simulink model "LCK"  (R2018b)
settings: Solver=FixedStepDiscrete  StartTime=0.0  StopTime=inf  FixedStep=0.01  RelTol=1e-3
PostLoadFcn:
  | if any(exist('dsrtsu_mdlpostloadfcn', 'file') ~= 0), dsrtsu_mdlpostloadfcn('Execute', bdroot); end
values from neighbouring files (symbols this model uses):
  C_DEG2RAD = 0.0175    [LCK_Macro.sldd]
  C_KPH2MPS = 0.2778    [LCK_Macro.sldd]
  C_NEARZERO = 0.0001    [LCK_Macro.sldd]
  C_ONE = 1.0    [LCK_Macro.sldd]
  C_RAD2DEG = 57.2958    [LCK_Macro.sldd]
  C_ZERO = 0.0    [LCK_Macro.sldd]
  k_accel_pedal_pos_per_speed_x : value not decoded    [LCK_LogicPara.sldd]
  k_accel_pedal_pos_per_speed_z : value not decoded    [LCK_LogicPara.sldd]
  k_brake_suprress_hold = 1000.0    [LCK_LogicPara.sldd]
  k_driver_appl_torque_filt = 50.0    [LCK_LogicPara.sldd]
  k_driver_suppression_hold_time = 3000.0    [LCK_LogicPara.sldd]
  k_hands_on_wheel_hold_msec = 500.0    [LCK_LogicPara.sldd]
  k_hands_on_wheel_torque_hi = 0.2    [LCK_LogicPara.sldd]
  k_hands_on_wheel_torque_lo = 0.15    [LCK_LogicPara.sldd]
  k_handsoff_delay_cycles = 50.0    [LCK_LogicPara.sldd]
  k_handsoff_torq_Lo_CR = 0.3    [LCK_LogicPara.sldd]
  k_handson_delay_cycles = 5.0    [LCK_LogicPara.sldd]
  k_HighAccel_suppress_hold = 3000.0    [LCK_LogicPara.sldd]
  k_HLR_suprress_hold = 3000.0    [LCK_LogicPara.sldd]
  k_hs_StrAng_CR_threshold_z : value not decoded    [LCK_LogicPara.sldd]
  k_LC_Exit_Switch = 0.0    [LCK_LogicPara.sldd]
  k_LCG_Configured = 1.0    [LCK_LogicPara.sldd]
  k_LCK_A0_Rdy2Act_UseConst = 0.0    [LCK_LogicPara.sldd]
  k_LCK_A0Fac_ActSta : value not decoded    [LCK_CtrlPara.sldd]
  k_LCK_A0Fac_DrvStm : value not decoded    [LCK_CtrlPara.sldd]
  k_LCK_A0Shift_LftCurv : value not decoded    [LCK_CtrlPara.sldd]
  k_LCK_A0Shift_RgtCurv : value not decoded    [LCK_CtrlPara.sldd]
  k_LCK_A0Shift_StraLan = 0.0    [LCK_CtrlPara.sldd]
  k_LCK_A0ShiftFac_Dy_LftCurv : value not decoded    [LCK_CtrlPara.sldd]
  k_LCK_A0ShiftFac_Dy_RgtCurv : value not decoded    [LCK_CtrlPara.sldd]
  k_LCK_A0ShiftFac_Vspd : value not decoded    [LCK_CtrlPara.sldd]
  k_LCK_accel_inhibit_thold = 35.0    [LCK_LogicPara.sldd]
  k_LCK_Active2Ready_Mask = 255.0    [LCK_LogicPara.sldd]
  k_LCK_CvatRateBks : value not decoded    [LCK_CtrlPara.sldd]
  k_LCK_CvatrBks : value not decoded    [LCK_CtrlPara.sldd]
  k_LCK_DFac_Dy : value not decoded    [LCK_CtrlPara.sldd]
  k_LCK_DFac_Dy_Curv : value not decoded    [LCK_CtrlPara.sldd]
  k_LCK_DFac_HaCurCen : value not decoded    [LCK_CtrlPara.sldd]
  k_LCK_DFac_HaCurSid : value not decoded    [LCK_CtrlPara.sldd]
  k_LCK_DFac_HadCurCen : value not decoded    [LCK_CtrlPara.sldd]
  k_LCK_DFac_HadCurSid : value not decoded    [LCK_CtrlPara.sldd]
  k_LCK_DFac_HadStrCen : value not decoded    [LCK_CtrlPara.sldd]
  k_LCK_DFac_HadStrSid : value not decoded    [LCK_CtrlPara.sldd]
  k_LCK_DFac_HaStrCen : value not decoded    [LCK_CtrlPara.sldd]
  k_LCK_DFac_HaStrSid : value not decoded    [LCK_CtrlPara.sldd]
  k_LCK_DFac_Rad : value not decoded    [LCK_CtrlPara.sldd]
  k_LCK_DFac_SA_CurCen : value not decoded    [LCK_CtrlPara.sldd]
  k_LCK_DFac_SA_CurSid : value not decoded    [LCK_CtrlPara.sldd]
  k_LCK_DFac_SA_StrCen : value not decoded    [LCK_CtrlPara.sldd]
  k_LCK_DFac_SA_StrSid : value not decoded    [LCK_CtrlPara.sldd]
  k_LCK_DFac_SS_CurCen : value not decoded    [LCK_CtrlPara.sldd]
  k_LCK_DFac_SS_CurSid : value not decoded    [LCK_CtrlPara.sldd]
  k_LCK_DFac_SS_StrCen : value not decoded    [LCK_CtrlPara.sldd]
  k_LCK_DFac_SS_StrSid : value not decoded    [LCK_CtrlPara.sldd]
  k_LCK_DFac_Vspd : value not decoded    [LCK_CtrlPara.sldd]
  k_LCK_DlyTm_DrvStim = 0.2    [LCK_CtrlPara.sldd]
  k_LCK_DTermMax = 2.0    [LCK_CtrlPara.sldd]
  k_LCK_DyBks_Curv : value not decoded    [LCK_CtrlPara.sldd]
  k_LCK_Enable_POOnly = 1.0    [LCK_LogicPara.sldd]
  k_LCK_Entry_DistBuffer = 0.1    [LCK_LogicPara.sldd]
  k_LCK_Fac_Vspd2RngThr_FalRec = 0.23    [LCK_CtrlPara.sldd]
  k_LCK_Ffw_CvatSwh = 0.0    [LCK_CtrlPara.sldd]
  k_LCK_Ffw_DyBks : value not decoded    [LCK_CtrlPara.sldd]
  k_LCK_Ffw_TimCon_CmdFlt = 0.0    [LCK_CtrlPara.sldd]
  k_LCK_FfwDeltaFac_Rad_Lft : value not decoded    [LCK_CtrlPara.sldd]
  k_LCK_FfwDeltaFac_Rad_Rgt : value not decoded    [LCK_CtrlPara.sldd]
  k_LCK_FfwDeltaFac_Vspd : value not decoded    [LCK_CtrlPara.sldd]
  k_LCK_FfwFac_CvatRate_Lft : value not decoded    [LCK_CtrlPara.sldd]
  k_LCK_FfwFac_CvatRate_Rgt : value not decoded    [LCK_CtrlPara.sldd]
  k_LCK_FfwFac_Dy : value not decoded    [LCK_CtrlPara.sldd]
  k_LCK_FfwFac_Rad_Lft : value not decoded    [LCK_CtrlPara.sldd]
  k_LCK_FfwFac_Rad_Rgt : value not decoded    [LCK_CtrlPara.sldd]
  k_LCK_FfwFac_Vspd : value not decoded    [LCK_CtrlPara.sldd]
  k_LCK_FfwTorq_Cvat : value not decoded    [LCK_CtrlPara.sldd]
  k_LCK_HAFac_ActSta : value not decoded    [LCK_CtrlPara.sldd]
  k_LCK_HAFac_DrvStm : value not decoded    [LCK_CtrlPara.sldd]
  k_LCK_HaloTime = 2000.0    [LCK_LogicPara.sldd]
  k_LCK_HaloTime_Switch = 0.0    [LCK_LogicPara.sldd]
  k_LCK_HARFac_ActSta : value not decoded    [LCK_CtrlPara.sldd]
  k_LCK_HARFac_DrvStm : value not decoded    [LCK_CtrlPara.sldd]
  k_LCK_Hed_DyBks : value not decoded    [LCK_CtrlPara.sldd]
  k_LCK_HedAngDiffX : value not decoded    [LCK_CtrlPara.sldd]
  k_LCK_HedAngRateDiffX : value not decoded    [LCK_CtrlPara.sldd]
  k_LCK_HndsOnWhel_DlyTm_Idl2Rdy = 0.0    [LCK_LogicPara.sldd]
  k_LCK_host_veh_width = 1.86    [LCK_LogicPara.sldd]
  k_LCK_Idle2Ready_Mask = 239.0    [LCK_LogicPara.sldd]
  k_LCK_Junc_SusTime = 1.0    [LCK_LogicPara.sldd]
  k_LCK_KpKdDecSlopeLmt = 10.0    [LCK_CtrlPara.sldd]
  k_LCK_KpKdIncSlopeLmt = 5.0    [LCK_CtrlPara.sldd]
  k_LCK_Lat_Ctrl_DFac_Lft = 1.0    [LCK_CtrlPara.sldd]
  k_LCK_Lat_Ctrl_DFac_Rgt = 1.05    [LCK_CtrlPara.sldd]
  k_LCK_Lat_Ctrl_Kd = 0.8    [LCK_CtrlPara.sldd]
  k_LCK_Lat_Ctrl_Ki = 0.5    [LCK_CtrlPara.sldd]
  k_LCK_Lat_Ctrl_Kp = 0.7    [LCK_CtrlPara.sldd]
  k_LCK_Lat_Ctrl_Kp_NearGain = 0.7    [LCK_CtrlPara.sldd]
  k_LCK_Lat_Ctrl_PFac_Lft = 1.0    [LCK_CtrlPara.sldd]
  k_LCK_Lat_Ctrl_PFac_Rgt = 1.05    [LCK_CtrlPara.sldd]
  k_LCK_Lat_Ctrl_TimCon_CmdFlt = 5.0    [LCK_CtrlPara.sldd]
  k_LCK_Lat_DFac_Rad : value not decoded    [LCK_CtrlPara.sldd]
  k_LCK_Lat_DFac_SS_Cur : value not decoded    [LCK_CtrlPara.sldd]
  k_LCK_Lat_DFac_SS_Str : value not decoded    [LCK_CtrlPara.sldd]
  k_LCK_Lat_DFac_Vspd : value not decoded    [LCK_CtrlPara.sldd]
  k_LCK_Lat_DyBks : value not decoded    [LCK_CtrlPara.sldd]
  k_LCK_Lat_IFac_Rad : value not decoded    [LCK_CtrlPara.sldd]
  k_LCK_Lat_IFac_Vspd : value not decoded    [LCK_CtrlPara.sldd]
  k_LCK_Lat_ILmtFac_Dy_CurvLan : value not decoded    [LCK_CtrlPara.sldd]
  k_LCK_Lat_ILmtFac_Dy_StraLan : value not decoded    [LCK_CtrlPara.sldd]
  k_LCK_Lat_ILmtFac_Rad : value not decoded    [LCK_CtrlPara.sldd]
  k_LCK_Lat_ILmtFac_Rad_NearGain = 1.0    [LCK_CtrlPara.sldd]
  k_LCK_Lat_ILmtFac_Vspd_CurvLan : value not decoded    [LCK_CtrlPara.sldd]
  k_LCK_Lat_ILmtFac_Vspd_StraLan : value not decoded    [LCK_CtrlPara.sldd]
  k_LCK_Lat_ITermLmt_Dy = 1.0    [LCK_CtrlPara.sldd]
  k_LCK_Lat_KpKdDecSlopeLmt = 10.0    [LCK_CtrlPara.sldd]
  k_LCK_Lat_KpKdIncSlopeLmt = 10.0    [LCK_CtrlPara.sldd]
  k_LCK_Lat_PFac_Dy_InnLftCur : value not decoded    [LCK_CtrlPara.sldd]
  k_LCK_Lat_PFac_Dy_InnRgtCur : value not decoded    [LCK_CtrlPara.sldd]
  k_LCK_Lat_PFac_Dy_OutLftCur : value not decoded    [LCK_CtrlPara.sldd]
  k_LCK_Lat_PFac_Dy_OutRgtCur : value not decoded    [LCK_CtrlPara.sldd]
  k_LCK_Lat_PFac_Dy_Str : value not decoded    [LCK_CtrlPara.sldd]
  k_LCK_Lat_PFac_Rad : value not decoded    [LCK_CtrlPara.sldd]
  ... (+153 more)
undefined symbols (not defined in the file or in its folder): k_LCK_CurvBks, K_LCK_SPA0A1A2_LMRngCmp_y
libraries: LateralControl_fcns_lib x59, simulink x24
(part 38 of 47)

== system LCK/Lateral_Control_Module/Adas_Lateral_Control_LCK_Core/Module 8/Module 0/Definition  Limit ==
  Road_Radius : Inport
  Vspd : Inport  Port=2
  Dy_1 : Inport  Port=3
  Str_Flag : Inport  Port=4
  Abs : Abs
  Add : Sum
  Constant : Constant  OutDataTypeStr=single
  Divide : Product  Inputs=*/
  Product1 : Product  Inputs=4
  Product2 : Product  Inputs=4
  Product7 : Product
  Switch4 : Switch  Criteria=u2 > Threshold
  Switch5 : Switch  Criteria=u2 > Threshold
  k_LCK_Lat_ILmtFac_Dy_CurvLan : Lookup_n-D  NumberOfTableDimensions=1  BreakpointsForDimension1=k_LCK_Lat_DyBks  IndexSearchMethod=Linear search  Table=k_LCK_Lat_ILmtFac_Dy_CurvLan  ExtrapMethod=Clip  InternalRulePriority=Speed  RndMeth=Simplest  InputSameDT=on
  k_LCK_Lat_ILmtFac_Dy_StraLan : Lookup_n-D  NumberOfTableDimensions=1  BreakpointsForDimension1=k_LCK_Lat_DyBks  IndexSearchMethod=Linear search  Table=k_LCK_Lat_ILmtFac_Dy_StraLan  ExtrapMethod=Clip  InternalRulePriority=Speed  RndMeth=Simplest  InputSameDT=on
  k_LCK_Lat_ILmtFac_Rad : Lookup_n-D  NumberOfTableDimensions=1  BreakpointsForDimension1=k_LCK_RadBks  IndexSearchMethod=Linear search  Table=k_LCK_Lat_ILmtFac_Rad  ExtrapMethod=Clip  InternalRulePriority=Speed  RndMeth=Simplest  InputSameDT=on
  k_LCK_Lat_ILmtFac_Rad_NearGain : Constant  Value=k_LCK_Lat_ILmtFac_Rad_NearGain
  k_LCK_Lat_ILmtFac_Vspd_CurvLan : Lookup_n-D  NumberOfTableDimensions=1  BreakpointsForDimension1=k_LCK_VspdBks  IndexSearchMethod=Linear search  Table=k_LCK_Lat_ILmtFac_Vspd_CurvLan  ExtrapMethod=Clip  InternalRulePriority=Speed  RndMeth=Simplest  InputSameDT=on
  k_LCK_Lat_ILmtFac_Vspd_StraLan : Lookup_n-D  NumberOfTableDimensions=1  BreakpointsForDimension1=k_LCK_VspdBks  IndexSearchMethod=Linear search  Table=k_LCK_Lat_ILmtFac_Vspd_StraLan  ExtrapMethod=Clip  InternalRulePriority=Speed  RndMeth=Simplest  InputSameDT=on
  k_LCK_Lat_ITermLmt_Dy : Constant  Value=k_LCK_Lat_ITermLmt_Dy
  ITerm_Limit_1 : Outport
  ITerm_Limit_0 : Outport  Port=2
  wires:
  Vspd/1 -> k_LCK_Lat_ILmtFac_Vspd_CurvLan/1, k_LCK_Lat_ILmtFac_Vspd_StraLan/1
  k_LCK_Lat_ILmtFac_Vspd_CurvLan/1 -> Switch5/3
  Str_Flag/1 -> Switch5/2, Switch4/2
  k_LCK_Lat_ILmtFac_Vspd_StraLan/1 -> Switch5/1
  k_LCK_Lat_ILmtFac_Dy_CurvLan/1 -> Switch4/3
  k_LCK_Lat_ILmtFac_Dy_StraLan/1 -> Switch4/1
  Road_Radius/1 -> k_LCK_Lat_ILmtFac_Rad/1
  Dy_1/1 -> Abs/1
  Switch4/1 -> Product2/2, Product1/1
  Switch5/1 -> Product2/3, Product1/2
  k_LCK_Lat_ITermLmt_Dy/1 -> Product2/1, Product1/4
  Product2/1 -> ITerm_Limit_0/1
  Product1/1 -> ITerm_Limit_1/1
  Abs/1 -> k_LCK_Lat_ILmtFac_Dy_StraLan/1, k_LCK_Lat_ILmtFac_Dy_CurvLan/1
  k_LCK_Lat_ILmtFac_Rad_NearGain/1 -> Product7/2, Add/2
  Constant/1 -> Add/1
  k_LCK_Lat_ILmtFac_Rad/1 -> Divide/1
  Add/1 -> Divide/2
  Divide/1 -> Product1/3, Product7/1
  Product7/1 -> Product2/4

== system LCK/Lateral_Control_Module/Adas_Lateral_Control_LCK_Core/Module 8/Module 0/Definition Fac 2 ==
  Dy_0 : Inport
  Str_Flag : Inport  Port=2
  Inn_Cur_Flag_0 : Inport  Port=3
  Cur_Flag : Inport  Port=4
  Abs : Abs
  Switch{3,10,12..13} (4 alike) : Switch  Criteria=u2 > Threshold
  k_LCK_Lat_PFac_Dy_InnLftCur : Lookup_n-D  NumberOfTableDimensions=1  BreakpointsForDimension1=k_LCK_Lat_DyBks  IndexSearchMethod=Linear search  Table=k_LCK_Lat_PFac_Dy_InnLftCur  ExtrapMethod=Clip  InternalRulePriority=Speed  RndMeth=Simplest  InputSameDT=on
  k_LCK_Lat_PFac_Dy_InnRgtCur : Lookup_n-D  NumberOfTableDimensions=1  BreakpointsForDimension1=k_LCK_Lat_DyBks  IndexSearchMethod=Linear search  Table=k_LCK_Lat_PFac_Dy_InnRgtCur  ExtrapMethod=Clip  InternalRulePriority=Speed  RndMeth=Simplest  InputSameDT=on
  k_LCK_Lat_PFac_Dy_OutLftCur : Lookup_n-D  NumberOfTableDimensions=1  BreakpointsForDimension1=k_LCK_Lat_DyBks  IndexSearchMethod=Linear search  Table=k_LCK_Lat_PFac_Dy_OutLftCur  ExtrapMethod=Clip  InternalRulePriority=Speed  RndMeth=Simplest  InputSameDT=on
  k_LCK_Lat_PFac_Dy_OutRgtCur : Lookup_n-D  NumberOfTableDimensions=1  BreakpointsForDimension1=k_LCK_Lat_DyBks  IndexSearchMethod=Linear search  Table=k_LCK_Lat_PFac_Dy_OutRgtCur  ExtrapMethod=Clip  InternalRulePriority=Speed  RndMeth=Simplest  InputSameDT=on
  k_LCK_Lat_PFac_Dy_Str : Lookup_n-D  NumberOfTableDimensions=1  BreakpointsForDimension1=k_LCK_Lat_DyBks  IndexSearchMethod=Linear search  Table=k_LCK_Lat_PFac_Dy_Str  ExtrapMethod=Clip  InternalRulePriority=Speed  RndMeth=Simplest  InputSameDT=on
  LatCtrl_P0Fac_Dy : Outport
  wires:
  k_LCK_Lat_PFac_Dy_OutLftCur/1 -> Switch10/3
  Inn_Cur_Flag_0/1 -> Switch13/2, Switch10/2
  k_LCK_Lat_PFac_Dy_InnLftCur/1 -> Switch10/1
  Switch10/1 -> Switch12/1
  Switch13/1 -> Switch12/3
  Dy_0/1 -> Abs/1
  Switch12/1 -> Switch3/3
  Cur_Flag/1 -> Switch12/2
  k_LCK_Lat_PFac_Dy_OutRgtCur/1 -> Switch13/3
  k_LCK_Lat_PFac_Dy_InnRgtCur/1 -> Switch13/1
  k_LCK_Lat_PFac_Dy_Str/1 -> Switch3/1
  Str_Flag/1 -> Switch3/2
  Switch3/1 -> LatCtrl_P0Fac_Dy/1
  Abs/1 -> k_LCK_Lat_PFac_Dy_Str/1, k_LCK_Lat_PFac_Dy_OutRgtCur/1, k_LCK_Lat_PFac_Dy_InnRgtCur/1, k_LCK_Lat_PFac_Dy_OutLftCur/1, k_LCK_Lat_PFac_Dy_InnLftCur/1

== system LCK/Lateral_Control_Module/Adas_Lateral_Control_LCK_Core/Module 8/Module 0/Definition Fac 3 ==
  Cur_Flag : Inport
  Inn_Cur_Flag_1 : Inport  Port=2
  Dy_1 : Inport  Port=3
  Str_Flag : Inport  Port=4
  Abs : Abs
  Switch{3,10,12..13} (4 alike) : Switch  Criteria=u2 > Threshold
  k_LCK_Lat_PFac_Dy_InnLftCur : Lookup_n-D  NumberOfTableDimensions=1  BreakpointsForDimension1=k_LCK_Lat_DyBks  IndexSearchMethod=Linear search  Table=k_LCK_Lat_PFac_Dy_InnLftCur  ExtrapMethod=Clip  InternalRulePriority=Speed  RndMeth=Simplest  InputSameDT=on
  k_LCK_Lat_PFac_Dy_InnRgtCur : Lookup_n-D  NumberOfTableDimensions=1  BreakpointsForDimension1=k_LCK_Lat_DyBks  IndexSearchMethod=Linear search  Table=k_LCK_Lat_PFac_Dy_InnRgtCur  ExtrapMethod=Clip  InternalRulePriority=Speed  RndMeth=Simplest  InputSameDT=on
  k_LCK_Lat_PFac_Dy_OutLftCur : Lookup_n-D  NumberOfTableDimensions=1  BreakpointsForDimension1=k_LCK_Lat_DyBks  IndexSearchMethod=Linear search  Table=k_LCK_Lat_PFac_Dy_OutLftCur  ExtrapMethod=Clip  InternalRulePriority=Speed  RndMeth=Simplest  InputSameDT=on
  k_LCK_Lat_PFac_Dy_OutRgtCur : Lookup_n-D  NumberOfTableDimensions=1  BreakpointsForDimension1=k_LCK_Lat_DyBks  IndexSearchMethod=Linear search  Table=k_LCK_Lat_PFac_Dy_OutRgtCur  ExtrapMethod=Clip  InternalRulePriority=Speed  RndMeth=Simplest  InputSameDT=on
  k_LCK_Lat_PFac_Dy_Str : Lookup_n-D  NumberOfTableDimensions=1  BreakpointsForDimension1=k_LCK_Lat_DyBks  IndexSearchMethod=Linear search  Table=k_LCK_Lat_PFac_Dy_Str  ExtrapMethod=Clip  InternalRulePriority=Speed  RndMeth=Simplest  InputSameDT=on
  LatCtrl_P1Fac_Dy : Outport
  wires:
  Abs/1 -> k_LCK_Lat_PFac_Dy_InnLftCur/1, k_LCK_Lat_PFac_Dy_OutLftCur/1, k_LCK_Lat_PFac_Dy_InnRgtCur/1, k_LCK_Lat_PFac_Dy_OutRgtCur/1, k_LCK_Lat_PFac_Dy_Str/1
  Switch3/1 -> LatCtrl_P1Fac_Dy/1
  Str_Flag/1 -> Switch3/2
  k_LCK_Lat_PFac_Dy_Str/1 -> Switch3/1
  k_LCK_Lat_PFac_Dy_InnRgtCur/1 -> Switch13/1
  k_LCK_Lat_PFac_Dy_OutRgtCur/1 -> Switch13/3
  Cur_Flag/1 -> Switch12/2
  Switch12/1 -> Switch3/3
  Dy_1/1 -> Abs/1
  Switch13/1 -> Switch12/3
  Switch10/1 -> Switch12/1
  k_LCK_Lat_PFac_Dy_InnLftCur/1 -> Switch10/1
  Inn_Cur_Flag_1/1 -> Switch10/2, Switch13/2
  k_LCK_Lat_PFac_Dy_OutLftCur/1 -> Switch10/3

== system LCK/Lateral_Control_Module/Adas_Lateral_Control_LCK_Core/Module 8/Module 0/Definition Fac 4 ==
  Vspd : Inport
  k_LCK_Lat_DFac_Vspd : Lookup_n-D  NumberOfTableDimensions=1  BreakpointsForDimension1=k_LCK_VspdBks  IndexSearchMethod=Linear search  Table=k_LCK_Lat_DFac_Vspd  ExtrapMethod=Clip  InternalRulePriority=Speed  RndMeth=Simplest  InputSameDT=on
  k_LCK_Lat_IFac_Vspd : Lookup_n-D  NumberOfTableDimensions=1  BreakpointsForDimension1=k_LCK_VspdBks  IndexSearchMethod=Linear search  Table=k_LCK_Lat_IFac_Vspd  ExtrapMethod=Clip  InternalRulePriority=Speed  RndMeth=Simplest  InputSameDT=on
  k_LCK_Lat_PFac_Vspd : Lookup_n-D  NumberOfTableDimensions=1  BreakpointsForDimension1=k_LCK_VspdBks  IndexSearchMethod=Linear search  Table=k_LCK_Lat_PFac_Vspd  ExtrapMethod=Clip  InternalRulePriority=Speed  RndMeth=Simplest  InputSameDT=on
  LatCtrl_PFac_Vspd : Outport
  LatCtrl_IFac_Vspd : Outport  Port=2
  LatCtrl_DFac_Vspd : Outport  Port=3
  wires:
  k_LCK_Lat_PFac_Vspd/1 -> LatCtrl_PFac_Vspd/1
  Vspd/1 -> k_LCK_Lat_PFac_Vspd/1, k_LCK_Lat_IFac_Vspd/1, k_LCK_Lat_DFac_Vspd/1
  k_LCK_Lat_IFac_Vspd/1 -> LatCtrl_IFac_Vspd/1
  k_LCK_Lat_DFac_Vspd/1 -> LatCtrl_DFac_Vspd/1
